simulink model "Planta_26_3_prueba_ciclodoble"  (R2021a)
settings: Solver=VariableStepAuto  StartTime=0.0  StopTime=300  MaxStep=1e-2  RelTol=1e-3
values from neighbouring files (symbols this model uses):
  alfahmax = ((2*ahmax)/(rhd))    (= 2)    [valoresPlanta_29_9_24.m]    (also in valoresPlanta_V3.m; valoresPlanta_v4.m)
  alfatmax = atmax/rtd    (= 1.6)    [valoresPlanta_29_9_24.m]    (also in valoresPlanta_V3.m; valoresPlanta_v4.m)
  atmax = 0.8    [valoresPlanta_29_9_24.m]    (also in valoresPlanta_V3.m; valoresPlanta_v4.m)
  ax_max = 0.8    [valoresPlanta_29_9_24.m]    (also in valoresPlanta_v4.m)
  ay_max = 0.75    [valoresPlanta_29_9_24.m]    (also in valoresPlanta_v4.m)
  bcx = 1e6    (= 1000000)    [Valores_1.m]    (also in valoresPlanta.m; valoresPlanta_29_9_24.m; valoresPlanta_V3.m; valoresPlanta_v4.m)
  bcy = 1e7    (= 10000000)    [Valores_1.m]    (also in valoresPlanta.m; valoresPlanta_29_9_24.m; valoresPlanta_V3.m; valoresPlanta_v4.m)
  bh_eq = bhm*ih^2+bhd    (= 8720)    [Valores.m]    (also in Valores_1.m; valoresPlanta.m; valoresPlanta_29_9_24.m; valoresPlanta_V3.m)
  bhb = 1e8    (= 100000000)    [Valores.m]    (also in Valores_1.m; valoresPlanta.m; valoresPlanta_29_9_24.m; valoresPlanta_V3.m)
  bhEb = 2.2e9    (= 2200000000)    [Valores.m]    (also in Valores_1.m; valoresPlanta.m; valoresPlanta_29_9_24.m; valoresPlanta_V3.m)
  bt = 90.0    (= 90)    [Valores.m]    (also in Valores_1.m; valoresPlanta.m; valoresPlanta_29_9_24.m; valoresPlanta_V3.m)
  bt_eq = btd+(btm*(it^2))    (= 5401.8)    [valoresPlanta.m]    (also in valoresPlanta_29_9_24.m; valoresPlanta_V3.m; valoresPlanta_v4.m)
  btb = 5e6    (= 5000000)    [Valores.m]    (also in Valores_1.m; valoresPlanta.m; valoresPlanta_29_9_24.m; valoresPlanta_V3.m)
  btw = 3.0e3    (= 3000)    [Valores.m]    (also in Valores_1.m; valoresPlanta.m; valoresPlanta_29_9_24.m; valoresPlanta_V3.m)
  bwu = 150    [Valores.m]    (also in Valores_1.m; valoresPlanta.m; valoresPlanta_29_9_24.m; valoresPlanta_V3.m)
  estado_cont = [x_positions; hy_cont]    [perfilObsaculos.m]    (also in valoresPlanta_29_9_24.m = [x_positions; [hy_muelle hy_cont]]; valoresPlanta_v4.m = [x_positions; [hy_muelle hy_cont]])
  g = 9.80665    [Valores.m]    (also in Valores_1.m; valoresPlanta.m; valoresPlanta_29_9_24.m; valoresPlanta_V3.m)
  Hc = 0    [Valores.m]    (also in Valores_1.m = 2.5; valoresPlanta.m = 2.5; valoresPlanta_29_9_24.m = 2.5; valoresPlanta_V3.m = 2.5)
  hx_cont = 2.5    [perfilObsaculos.m]    (also in puntosTrayectoria.m; valoresPlanta_29_9_24.m; valoresPlanta_v4.m)
  ih = 22    [Valores.m]    (also in Valores_1.m; valoresPlanta.m; valoresPlanta_29_9_24.m; valoresPlanta_V3.m)
  it = 30    [Valores.m]    (also in Valores_1.m; valoresPlanta.m; valoresPlanta_29_9_24.m; valoresPlanta_V3.m)
  Jh_eq = Jhm_hb*ih^2+Jhd_hEb    (= 18320)    [Valores.m]    (also in Valores_1.m; valoresPlanta.m; valoresPlanta_29_9_24.m; valoresPlanta_V3.m)
  Jt_eq = Jtd+(Jtm_tb*(it^2))    (= 7500)    [valoresPlanta.m]    (also in valoresPlanta_29_9_24.m; valoresPlanta_V3.m; valoresPlanta_v4.m)
  kcy = 1.8e9    (= 1800000000)    [Valores_1.m]    (also in valoresPlanta.m; valoresPlanta_29_9_24.m; valoresPlanta_V3.m; valoresPlanta_v4.m)
  KDh = Jeq2 * w_posh^3    (= -12245.4404091)    [Valores.m]    (also in Valores_1.m = Jeq2 * w_posh; valoresPlanta.m = Jeq2 * w_posh; valoresPlanta_29_9_24.m = Jh_eq * n * w_posh; valoresPlanta_V3.m = Jeq2 * w_posh)
  KDt = Meq2 * w_post^3    (= -4728.86946035)    [Valores.m]    (also in Valores_1.m = Meq2 * w_post; valoresPlanta.m = Meq2 * w_post; valoresPlanta_29_9_24.m = 10127; valoresPlanta_V3.m = Meq2 * w_post)
  KIh = Jeq2 * w_posh^2    (= 2572.66592082)    [Valores.m]    (also in Valores_1.m = Jeq2 * w_posh^3; valoresPlanta.m = Jeq2 * w_posh^3; valoresPlanta_29_9_24.m = Jh_eq * w_posh^3; valoresPlanta_V3.m = Jeq2 * w_posh^3)
  KIt = Meq2 * w_post^2    (= 1307.690244)    [Valores.m]    (also in Valores_1.m = Meq2 * w_post^3; valoresPlanta.m = Meq2 * w_post^3; valoresPlanta_29_9_24.m = 6809.6; valoresPlanta_V3.m = Meq2 * w_post^3)
  KPh = Jeq2 * w_posh    (= -540.495867769)    [Valores.m]    (also in Valores_1.m = Jeq2 * w_posh^2; valoresPlanta.m = Jeq2 * w_posh^2; valoresPlanta_29_9_24.m = Jh_eq * n * w_posh^2; valoresPlanta_V3.m = Jeq2 * w_posh^2)
  KPt = Meq2 * w_post    (= -361.62)    [Valores.m]    (also in Valores_1.m = Meq2 * w_post^2; valoresPlanta.m = Meq2 * w_post^2; valoresPlanta_29_9_24.m = 14123; valoresPlanta_V3.m = Meq2 * w_post^2)
  Ktw = 4.8e5    (= 480000)    [Valores.m]    (also in Valores_1.m; valoresPlanta.m; valoresPlanta_29_9_24.m; valoresPlanta_V3.m)
  kwu = 2.36e8    (= 236000000)    [Valores.m]    (also in Valores_1.m; valoresPlanta.m; valoresPlanta_29_9_24.m; valoresPlanta_V3.m)
  Mc_max = 5e4    (= 50000)    [Valores.m]    (also in Valores_1.m; valoresPlanta.m; valoresPlanta_29_9_24.m; valoresPlanta_V3.m)
  Mc_min = 2e3    (= 2000)    [Valores.m]    (also in Valores_1.m; valoresPlanta.m; valoresPlanta_29_9_24.m; valoresPlanta_V3.m)
  Meq = Mt+(it^2*Jtm_tb+Jtd)/rtd^2    (= 60000)    [Valores.m]    (also in Valores_1.m; valoresPlanta_29_9_24.m; valoresPlanta_v4.m)
  Mt = 30000    [Valores.m]    (also in Valores_1.m; valoresPlanta.m; valoresPlanta_29_9_24.m; valoresPlanta_V3.m)
  pos = [p0; p1; p2; p3; p4; p5]    [calcularTrayectoria2_prueba.m]    (also in perfilObsaculos.m = puntosTrayectoria(4, 1.5, 20, [-20,0], estado_cont, hy_cont,; puntosTrayectoria.m; valoresPlanta_29_9_24.m = calcularTrayectoria2_prueba(vx_max, vhmax, ax_max, Hc, hx_co; valoresPlanta_v4.m = calcularTrayectoria2_prueba(vx_max, vhmax, ax_max, Hc, hx_co)
  rhd = 0.75    [Valores.m]    (also in Valores_1.m; valoresPlanta.m; valoresPlanta_29_9_24.m; valoresPlanta_V3.m)
  rtd = 0.5    [Valores.m]    (also in Valores_1.m; valoresPlanta.m; valoresPlanta_29_9_24.m; valoresPlanta_V3.m)
  tau_hm = 1e-3    (= 0.001)    [valoresPlanta.m]    (also in valoresPlanta_29_9_24.m; valoresPlanta_V3.m; valoresPlanta_v4.m)
  tau_tm = 1e-3    (= 0.001)    [Valores.m]    (also in Valores_1.m; valoresPlanta.m; valoresPlanta_29_9_24.m; valoresPlanta_V3.m)
  Thb_Max = 5e4    (= 50000)    [Valores.m]    (also in Valores_1.m; valoresPlanta.m; valoresPlanta_29_9_24.m; valoresPlanta_V3.m)
  ThEb_Max = 1.1e6    (= 1100000)    [Valores.m]    (also in Valores_1.m; valoresPlanta.m; valoresPlanta_29_9_24.m; valoresPlanta_V3.m)
  Thm_Max = 2e4    (= 20000)    [Valores.m]    (also in Valores_1.m; valoresPlanta.m; valoresPlanta_29_9_24.m; valoresPlanta_V3.m)
  Ttb_Max = 5e3    (= 5000)    [Valores.m]    (also in Valores_1.m; valoresPlanta.m; valoresPlanta_29_9_24.m; valoresPlanta_V3.m)
  Ttm_Max = 3e3    (= 3000)    [Valores.m]    (also in Valores_1.m; valoresPlanta.m; valoresPlanta_29_9_24.m = 4000; valoresPlanta_V3.m)
  v_x_max = 4    [Valores_1.m]    (also in valoresPlanta.m; valoresPlanta_V3.m = 0.4)
  vhmax = 3    [valoresPlanta_29_9_24.m]    (also in valoresPlanta_V3.m; valoresPlanta_v4.m)
  vx_max = 4    [valoresPlanta_29_9_24.m]    (also in valoresPlanta_v4.m)
  whmMax = P/Thm_Max    (= 47.8075)    [Valores_1.m]    (also in valoresPlanta.m; valoresPlanta_29_9_24.m = 176; valoresPlanta_V3.m; valoresPlanta_v4.m)
  whmMin = 0.02    [valoresPlanta_29_9_24.m]    (also in valoresPlanta_v4.m = 0.2)
  wtmMax = (4/rtd)*it    (= 240)    [Valores_1.m]    (also in valoresPlanta.m; valoresPlanta_29_9_24.m; valoresPlanta_V3.m; valoresPlanta_v4.m)
  wtmMin = 0.02    [valoresPlanta_29_9_24.m]    (also in valoresPlanta_v4.m = 0.2)
  xLimMax = 49    [valoresPlanta_29_9_24.m]    (also in valoresPlanta_v4.m)
  xLimMin = -29    [valoresPlanta_29_9_24.m]    (also in valoresPlanta_v4.m)
  y0 = 2.5    [valoresPlanta_29_9_24.m]    (also in valoresPlanta_v4.m)
  yLimMax = 44    [valoresPlanta_29_9_24.m]    (also in valoresPlanta_v4.m)
  yLimMin = -19    [valoresPlanta_29_9_24.m]    (also in valoresPlanta_v4.m)
  Yt0 = 45    [Valores.m]    (also in Valores_1.m; valoresPlanta.m; valoresPlanta_29_9_24.m; valoresPlanta_V3.m)
undefined symbols (not defined in the file or in its folder): sigbuilder_block, x0
libraries: vrlib x1, simulink_extras x1, cstblocks x1, simulink x1
(part 3 of 3)

== matlab function Planta_26_3_prueba_ciclodoble/Control Supervisor/fcn ==
  data: Mc_Max input; Mcx output; Mc_Min input; flag_carga input
function Mcx = fcn(Mc_Max, Mc_Min, flag_carga)
%Agregar: sobrecarga
if (flag_carga == 1)
    Mcx = Mc_Min + (Mc_Max - Mc_Min)*rand(1);
    %ml = Mc_Max + 0.01 * randi([1,15],1) * Mc_Max;
else
    Mcx = 0;
end
end

== stateflow chart Planta_26_3_prueba_ciclodoble/Frenos Traslación ==
  state FrenosOperacion
    state BRKt_off
      during:
      Ttb=-btb*wtm;
      Ttb=min(Ttb_Max,max(-Ttb_Max, Ttb));
    state BRKt_on
      during:
      Ttb=0;
    (default) -> BRKt_off
    BRKt_off -> BRKt_on : [BRKt==1 ]
    BRKt_on -> BRKt_off : [BRKt==0]
  data: Ttb output; wtm input; btb parameter; BRKt input; Ttb_Max input

== stateflow chart Planta_26_3_prueba_ciclodoble/Chart ==
  state Masa
    entry:
    if (modo_tw == 1)
    Mcx = fcn(Mc_max, Mc_min);
    else
    Mcx = 0;
    end
  data: Mc_MAX function_input; Mc_MIN function_input; ML function_output; Mc_max parameter; Mcx output; Mc_min parameter; modo_tw input
  function ML = fcn(Mc_MAX, Mc_MIN):
    | function ML = fcn(Mc_MAX, Mc_MIN)
    | %Agregar: sobrecarga
    | %if (flag_carga == 1)
    |     ML = Mc_MIN + (Mc_MAX - Mc_MIN)*rand(1);
    |     %ml = Mc_Max + 0.01 * randi([1,15],1) * Mc_Max;
    | %else
    |  %   ML = 0;
    | %end
    | end

== stateflow chart Planta_26_3_prueba_ciclodoble/Frenos Izaje  ==
  state FrenosOperacion
    state BRKh_off
      during:
      Thb=-bhb*whm;
      Thb=min(Thb_Max,max(-Thb_Max,Thb ));
    state BRKh_on
      during:
      Thb=0;
    (default) -> BRKh_off
    BRKh_off -> BRKh_on [order 1] : [BRKh==1 && BRKhE==1]
    BRKh_on -> BRKh_off [order 1] : [BRKh==0 && BRKhE==1]
  state FrenosEmergencia
    state BRKhE_off
      during:
      ThEb=-bhEb*whd;
      ThEb=min(ThEb_Max,max(-ThEb_Max, ThEb));
    state BRKhE_on
      during:
      ThEb=0;
    (default) -> BRKhE_off
    BRKhE_off -> BRKhE_on : [BRKhE==1]
    BRKhE_on -> BRKhE_off [order 1] : [BRKhE==0]
  BRKh_on -> FrenosEmergencia [order 2] : [BRKhE==0]
  BRKh_off -> FrenosEmergencia [order 2] : [BRKhE==0]
  BRKhE_on -> FrenosOperacion [order 2] : [BRKhE==1]
  (default) -> FrenosEmergencia
  data: whm input; bhb parameter; BRKh input; bhEb parameter; BRKhE input; Thb output; ThEb output; Thb_Max parameter; ThEb_Max parameter; whd input

== stateflow chart Planta_26_3_prueba_ciclodoble/Chart1 ==
  state Balanceo
    during:
    [KP,KD,WN]=balanceo(Meq, Mt,ml,l,g);
    %[KP,KD,KI,WN]=balanceo(ml, Mt, g, l)
  (default) -> Balanceo
  data: MEQ function_input; mt function_input; Ml function_input; L function_input; G function_input; Kd function_output; Kp function_output; wn function_output; l input; ml input; KD output; KP output; g parameter; Meq parameter; WN output; Mt parameter
  function [Kd,Kp, wn]=balanceo(MEQ, mt,Ml,L,G):
    | function [Kd,Kp, wn]=balanceo(MEQ, mt,Ml,L,G)
    |     
    | %     Kd=(1+(L*(mt+Ml)))/(mt+Ml);
    | %     Kp=(2*0.7*wn)/(mt+Ml);
    | %     w=((mt*G/((mt+Ml)*L))^0.5);
    | %     Kd=(mt*G/w^2 + (mt+Ml)*L)/(Ml+mt);
    | %     Kp=2*0.7*(-(mt+Ml)*L/(Ml+mt)+Kd);
    |     
    |     %correccion agustin
    |     %wn=((mt*G)/(L*(mt+Ml)))^(0.5);
    |     %Kd = L - (mt*G)/((mt+Ml)*wn^2);
    |     %Kp = (2*z*wn)/(L-Kd);
    |     %correcion matias
    |     z = 0.9;
    |     wn=((MEQ*G)/(L*(MEQ+Ml)))^(0.5);
    |     wn = 1 * wn; %el mejor: 2
    |     Kd = ((-MEQ*G)/(wn^2) +(MEQ+Ml)*L)* 1/(mt+Ml);
    |     Kp = (2*z*wn)*((MEQ+Ml)* L - Kd*(mt+Ml))/(mt+Ml);
    | end
    |  
    | % function [kp,kd,ki,wn] = balanceo(Ml,mt,G,L)
    | %     xita=0.9;%0.7;
    | %     wn=(mt*G/((mt+Ml)*L))^(1/2);
    | %     kd=-(mt*G/((mt+Ml)*(wn^(3))));
    | %     kp=(kd*(2*xita*wn-wn)+l);
    | %     ki=wn^2*(1-xita)*kd;
    | % end

== stateflow chart Planta_26_3_prueba_ciclodoble/Chart2 ==
  state Balanceo
    during:
    [KP,KD,KI,WN]=balanceoPID(Meq, Mt,ml,l,g)
    %[KP,KD,KI,WN]=balanceo(ml, Mt, g, l)
  (default) -> Balanceo
  data: MEQ function_input; mt function_input; Ml function_input; L function_input; G function_input; Kd function_output; Kp function_output; Ki function_output; wn function_output; l input; ml input; KD output; KP output; g parameter; Meq parameter; WN output; Mt parameter; KI output
  function [Kd,Kp,Ki,wn]=balanceoPID(MEQ, mt,Ml,L,G):
    | function [Kd,Kp,Ki,wn]=balanceoPID(MEQ, mt,Ml,L,G)
    |     
    | %     Kd=(1+(L*(mt+Ml)))/(mt+Ml);
    | %     Kp=(2*0.7*wn)/(mt+Ml);
    | %     w=((mt*G/((mt+Ml)*L))^0.5);
    | %     Kd=(mt*G/w^2 + (mt+Ml)*L)/(Ml+mt);
    | %     Kp=2*0.7*(-(mt+Ml)*L/(Ml+mt)+Kd);
    |     
    |     %correccion agustin
    |     %wn=((mt*G)/(L*(mt+Ml)))^(0.5);
    |     %Kd = L - (mt*G)/((mt+Ml)*wn^2);
    |     %Kp = (2*z*wn)/(L-Kd);
    |     %correcion matias
    |     z = 0.7;
    |     wn=((MEQ*G)/(L*(MEQ+Ml)))^(0.5);
    |     wn = 1 * wn; %el mejor: 2
    |     Ki = ((wn^2)*(Meq*L + Ml*(L+Kd)- Kd*mt) - MEQ*G)/(Ml-mt);
    |     Kp = ((2*z*wn)*((MEQ* L) - Ml*(L+Kd)-(Kd*mt)))/(Ml-mt);
    |     Kd = ((-MEQ*G)/(wn^2) +(MEQ+Ml)*L)* 1/(mt+Ml);    %cambiar
    | end
    |  
    | % function [kp,kd,ki,wn] = balanceo(Ml,mt,G,L)
    | %     xita=0.9;%0.7;
    | %     wn=(mt*G/((mt+Ml)*L))^(1/2);
    | %     kd=-(mt*G/((mt+Ml)*(wn^(3))));
    | %     kp=(kd*(2*xita*wn-wn)+l);
    | %     ki=wn^2*(1-xita)*kd;
    | % end

== stateflow chart Planta_26_3_prueba_ciclodoble/Chart3 ==
  state Balanceo
    during:
    [KI,KP,WN]=balanceoPI(Meq, Mt,ml,l,g);
    %[KP,KD,KI,WN]=balanceo(ml, Mt, g, l)
  (default) -> Balanceo
  data: MEQ function_input; mt function_input; Ml function_input; L function_input; G function_input; Ki function_output; Kp function_output; wn function_output; l input; ml input; KP output; g parameter; Meq parameter; WN output; Mt parameter; KI output
  function [Ki,Kp, wn]=balanceoPI(MEQ, mt,Ml,L,G):
    | function [Ki,Kp,wn]=balanceoPI(MEQ, mt,Ml,L,G)
    | 
    |     z = 0.9;
    |     wn=((MEQ*G)/(L*(MEQ+Ml)))^(0.5);
    |     wn = 1 * wn; %el mejor: 2
    |     Ki = ((wn^2)* ((MEQ+Ml)*L)- MEQ*G)/(mt+Ml);
    |     Kp = (2*z*wn)*((MEQ+Ml)* L )/(mt+Ml);
    | end
